simulink model "PTTransmCU"  (Simulink 7.5)
settings: Solver=ode45  StartTime=0.0  StopTime=inf  RelTol=1e-3
libraries: simulink x12, CarMaker4SL x1
(part 3 of 3)

== system PTTransmCU/CarMaker/IPG Vehicle/PowerTrain/TCU Example/PTTransmCU_In/CreateBus TCU_Cfg Misc ==
  In : Inport
  BusCreator : BusCreator  Inputs=2
  Demux : Demux  Outputs=2
  Out : Outport
  wires:
  In/1 -> Demux/1
  BusCreator/1 -> Out/1
  Demux/1 -> BusCreator/1  "TCU_Cfg ClKind"
  Demux/2 -> BusCreator/2  "TCU_Cfg nGearBoxM"

== system PTTransmCU/CarMaker/IPG Vehicle/PowerTrain/TCU Example/TCU Example/Don't do anything ==
  GearBoxOut : Inport  OutDataType=sfix(16)  OutScaling=2^0
  ClutchOut : Inport  Port=2  OutDataType=sfix(16)  OutScaling=2^0
  Action Port : ActionPort  ActionType=elseif
  Signal Conversion : SignalConversion  ConversionOutput=Bus copy
  GearBoxOut1 : Outport  OutDataType=sfix(16)  OutScaling=2^0
  ClutchOut.Pos : Outport  Port=2  OutDataType=sfix(16)  OutScaling=2^0
  wires:
  GearBoxOut/1 -> Signal Conversion/1
  ClutchOut/1 -> ClutchOut.Pos/1
  Signal Conversion/1 -> GearBoxOut1/1

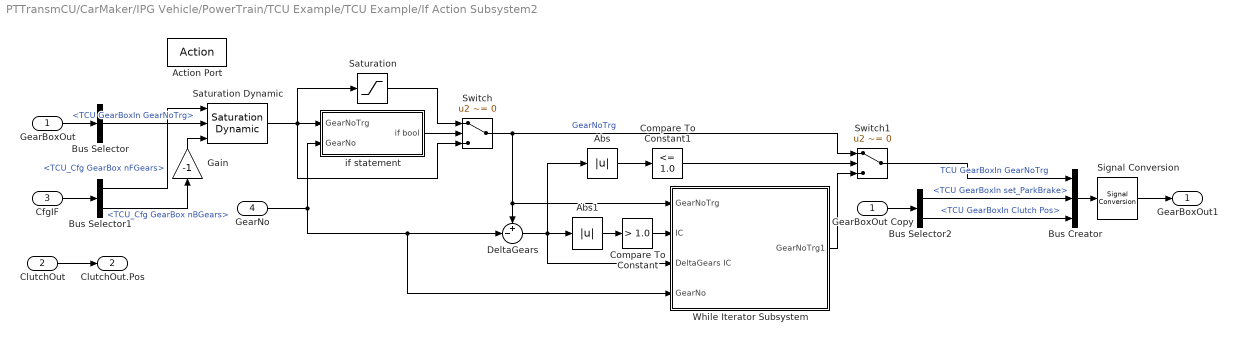
== system PTTransmCU/CarMaker/IPG Vehicle/PowerTrain/TCU Example/TCU Example/If Action Subsystem2 ==
  GearBoxOut : Inport  OutDataType=sfix(16)  OutScaling=2^0
  ClutchOut : Inport  Port=2  OutDataType=sfix(16)  OutScaling=2^0
  CfgIF : Inport  Port=3  OutDataType=sfix(16)  OutScaling=2^0
  GearNo : Inport  Port=4  OutDataType=sfix(16)  OutScaling=2^0
  Action Port : ActionPort  ActionType=else
  Abs : Abs  OutDataType=sfix(16)  OutScaling=2^0
  Abs1 : Abs  OutDataType=sfix(16)  OutScaling=2^0
  Bus Creator : BusCreator  Inputs=3
  Bus Selector : BusSelector  OutputSignals=TCU GearBoxIn GearNoTrg
  Bus Selector1 : BusSelector  OutputSignals=TCU_Cfg GearBox nFGears,TCU_Cfg GearBox nBGears
  Bus Selector2 : BusSelector  OutputSignals=TCU GearBoxIn set_ParkBrake,TCU GearBoxIn Clutch Pos
  Compare To Constant : simulink/Logic and Bit Operations/Compare To Constant  SystemSampleTime=-1  relop=>  const=1.0  LogicOutDataTypeMode=uint8  ZeroCross=off
  Compare To Constant1 : simulink/Logic and Bit Operations/Compare To Constant  SystemSampleTime=-1  relop=<=  const=1.0  LogicOutDataTypeMode=uint8  ZeroCross=off
  DeltaGears : Sum  Inputs=+-|  OutDataType=sfix(16)  OutScaling=2^-10
  Gain : Gain  Gain=-1  ParameterDataType=sfix(16)  ParameterScaling=2^0  OutDataType=sfix(16)  OutScaling=2^0
  GearBoxOut Copy : InportShadow  Port=1  OutDataType=sfix(16)  OutScaling=2^0
  Saturation : Saturate  UpperLimit=1  LowerLimit=-1  OutDataType=sfix(16)  OutScaling=2^0
  Saturation Dynamic : simulink/Discontinuities/Saturation Dynamic  SystemSampleTime=-1  OutMin=[]  OutMax=[]  OutDataTypeStr=Inherit: Same as second input  OutDataType=sfix(16)  OutScaling=2^-10  DoSatur=off
  Signal Conversion : SignalConversion  ConversionOutput=Bus copy
  Switch : Switch  Criteria=u2 ~= 0  OutDataType=sfix(16)  OutScaling=2^0
  Switch1 : Switch  Criteria=u2 ~= 0  Threshold=1  OutDataType=sfix(16)  OutScaling=2^0
  While Iterator Subsystem : Subsystem  TreatAsAtomicUnit=on
  if statement : Subsystem
  GearBoxOut1 : Outport  OutDataType=sfix(16)  OutScaling=2^0
  ClutchOut.Pos : Outport  Port=2  OutDataType=sfix(16)  OutScaling=2^0
  wires:
  GearBoxOut/1 -> Bus Selector/1
  Bus Selector/1 -> Saturation Dynamic/2  "<TCU GearBoxIn GearNoTrg>"
  CfgIF/1 -> Bus Selector1/1
  Bus Selector1/1 -> Saturation Dynamic/1  "<TCU_Cfg GearBox nFGears>"
  Bus Selector1/2 -> Gain/1  "<TCU_Cfg GearBox nBGears>"
  Gain/1 -> Saturation Dynamic/3
  ClutchOut/1 -> ClutchOut.Pos/1
  GearNo/1 -> if statement/2(GearNo), DeltaGears/2, While Iterator Subsystem/4(GearNo)
  Saturation Dynamic/1 -> if statement/1(GearNoTrg), Switch/3, Saturation/1
  if statement/1(if bool) -> Switch/2
  Saturation/1 -> Switch/1
  Switch/1 -> While Iterator Subsystem/1(GearNoTrg), DeltaGears/1, Switch1/1  "GearNoTrg"
  DeltaGears/1 -> Abs/1, While Iterator Subsystem/3(DeltaGears IC), Abs1/1
  Abs/1 -> Compare To Constant1/1
  Bus Creator/1 -> Signal Conversion/1
  Abs1/1 -> Compare To Constant/1
  Compare To Constant/1 -> While Iterator Subsystem/2(IC)
  Bus Selector2/2 -> Bus Creator/3  "<TCU GearBoxIn Clutch Pos>"
  Signal Conversion/1 -> GearBoxOut1/1
  Bus Selector2/1 -> Bus Creator/2  "<TCU GearBoxIn set_ParkBrake>"
  GearBoxOut Copy/1 -> Bus Selector2/1
  Compare To Constant1/1 -> Switch1/2
  While Iterator Subsystem/1(GearNoTrg1) -> Switch1/3
  Switch1/1 -> Bus Creator/1  "TCU GearBoxIn GearNoTrg"

== system PTTransmCU/CarMaker/IPG Vehicle/PowerTrain/TCU Example/TCU Example/Retrun Zero ==
  GearBoxOut : Inport  OutDataType=sfix(16)  OutScaling=2^0
  Action Port : ActionPort  ActionType=then
  Bus Creator : BusCreator  Inputs=3
  Bus Selector : BusSelector  OutputSignals=TCU GearBoxIn GearNoTrg,TCU GearBoxIn set_ParkBrake,TCU GearBoxIn Clutch Pos
  Constant : Constant  Value=1.0  OutDataType=sfix(16)  OutScaling=2^0
  Gain : Gain  Gain=0  ParameterDataType=sfix(16)  ParameterScaling=2^0  OutDataType=sfix(16)  OutScaling=2^0
  Gain1 : Gain  Gain=0  ParameterDataType=sfix(16)  ParameterScaling=2^0  OutDataType=sfix(16)  OutScaling=2^0
  Signal Conversion : SignalConversion  ConversionOutput=Bus copy
  GearBoxOut1 : Outport  OutDataType=sfix(16)  OutScaling=2^0
  ClutchOut.Pos : Outport  Port=2  OutDataType=sfix(16)  OutScaling=2^0  InitialOutput=1
  wires:
  Bus Selector/3 -> Bus Creator/3  "<TCU GearBoxIn Clutch Pos>"
  Bus Selector/2 -> Gain1/1  "<TCU GearBoxIn set_ParkBrake>"
  Bus Selector/1 -> Gain/1  "<TCU GearBoxIn GearNoTrg>"
  Gain/1 -> Bus Creator/1  "TCU GearBoxIn GearNoTrg"
  Gain1/1 -> Bus Creator/2  "TCU GearBoxIn set_ParkBrake"
  GearBoxOut/1 -> Bus Selector/1
  Constant/1 -> ClutchOut.Pos/1
  Bus Creator/1 -> Signal Conversion/1
  Signal Conversion/1 -> GearBoxOut1/1

== system PTTransmCU/CarMaker/IPG Vehicle/PowerTrain/TCU Example/TCU Example/If Action Subsystem2/While Iterator Subsystem ==
  GearNoTrg : Inport  OutDataType=sfix(16)  OutScaling=2^0
  IC : Inport  Port=2  OutDataType=sfix(16)  OutScaling=2^0
  DeltaGears IC : Inport  Port=3  OutDataType=sfix(16)  OutScaling=2^0
  GearNo : Inport  Port=4  OutDataType=sfix(16)  OutScaling=2^0
  Abs : Abs  OutDataType=sfix(16)  OutScaling=2^0
  Compare To Constant1 : simulink/Logic and Bit Operations/Compare To Constant  SystemSampleTime=-1  relop=>  const=1  LogicOutDataTypeMode=uint8  ZeroCross=off
  Constant : Constant  OutDataType=sfix(16)  OutScaling=2^0
  Constant1 : Constant  OutDataType=sfix(16)  OutScaling=2^0
  Sum : Sum  Inputs=|+-  OutDataType=sfix(16)  OutScaling=2^0
  Sum1 : Sum  Inputs=|-+  OutDataType=sfix(16)  OutScaling=2^0
  Sum2 : Sum  Inputs=++|  OutDataType=sfix(16)  OutScaling=2^0
  Switch : Switch  Criteria=u2 > Threshold  OutDataType=sfix(16)  OutScaling=2^0
  Unit Delay External IC : simulink/Additional Math & Discrete/Additional Discrete/Unit Delay External IC  SystemSampleTime=-1  tsamp=-1
  Unit Delay External IC1 : simulink/Additional Math & Discrete/Additional Discrete/Unit Delay External IC  SystemSampleTime=-1  tsamp=-1
  While Iterator : WhileIterator  MaxIters=-1  ResetStates=reset
  GearNoTrg1 : Outport  OutDataType=sfix(16)  OutScaling=2^0
  wires:
  IC/1 -> While Iterator/2
  Switch/1 -> GearNoTrg1/1, Unit Delay External IC/1, Sum/1
  Sum/1 -> Abs/1, Unit Delay External IC1/1
  Sum1/1 -> Switch/1
  Sum2/1 -> Switch/3
  Constant/1 -> Sum2/2
  Constant1/1 -> Sum1/1
  Unit Delay External IC/1 -> Sum1/2, Sum2/1
  GearNoTrg/1 -> Unit Delay External IC/2
  Abs/1 -> Compare To Constant1/1
  Compare To Constant1/1 -> While Iterator/1
  Unit Delay External IC1/1 -> Switch/2
  GearNo/1 -> Sum/2
  DeltaGears IC/1 -> Unit Delay External IC1/2

== system PTTransmCU/CarMaker/IPG Vehicle/PowerTrain/TCU Example/TCU Example/If Action Subsystem2/if statement ==
  GearNoTrg : Inport  OutDataType=sfix(16)  OutScaling=2^0
  GearNo : Inport  Port=2  OutDataType=sfix(16)  OutScaling=2^0
  Compare To Zero : simulink/Logic and Bit Operations/Compare To Zero  SystemSampleTime=-1  relop===  LogicOutDataTypeMode=uint8  ZeroCross=off
  Compare To Zero1 : simulink/Logic and Bit Operations/Compare To Zero  SystemSampleTime=-1  relop=>  LogicOutDataTypeMode=uint8  ZeroCross=off
  Compare To Zero2 : simulink/Logic and Bit Operations/Compare To Zero  SystemSampleTime=-1  relop=<  LogicOutDataTypeMode=uint8  ZeroCross=off
  Compare To Zero3 : simulink/Logic and Bit Operations/Compare To Zero  SystemSampleTime=-1  relop=<  LogicOutDataTypeMode=uint8  ZeroCross=off
  Compare To Zero4 : simulink/Logic and Bit Operations/Compare To Zero  SystemSampleTime=-1  relop=>  LogicOutDataTypeMode=uint8  ZeroCross=off
  Logical Operator : Logic  AllPortsSameDT=off  OutDataTypeMode=boolean  OutDataTypeStr=boolean
  Logical Operator1 : Logic  AllPortsSameDT=off  OutDataTypeMode=boolean  OutDataTypeStr=boolean
  Logical Operator2 : Logic  Operator=OR  Inputs=3  AllPortsSameDT=off  OutDataTypeMode=boolean  OutDataTypeStr=boolean
  if bool : Outport  OutDataType=sfix(16)  OutScaling=2^0
  wires:
  GearNo/1 -> Compare To Zero/1, Compare To Zero1/1, Compare To Zero3/1
  GearNoTrg/1 -> Compare To Zero2/1, Compare To Zero4/1
  Compare To Zero1/1 -> Logical Operator/1
  Compare To Zero2/1 -> Logical Operator/2
  Compare To Zero3/1 -> Logical Operator1/1
  Compare To Zero4/1 -> Logical Operator1/2
  Logical Operator2/1 -> if bool/1
  Compare To Zero/1 -> Logical Operator2/1
  Logical Operator/1 -> Logical Operator2/2
  Logical Operator1/1 -> Logical Operator2/3
